simulink model "stepRecovery"  (Simulink 8.7)
settings: Solver=FixedStepDiscrete  StartTime=0.0  StopTime="CONFIG.SIMULATION_TIME "  FixedStep=CONFIG.Ts  RelTol=1e-3
InitFcn:
  | cd(fileparts(which(bdroot)));
  | initStepRecovery;
values from neighbouring files (symbols this model uses):
  baseToWorldRotationPort = '/matlabTorqueBalancing/floatingBaseRotationMatrix:i'    [esperimento_fake2.mat]    (also in initStepRecovery.m = ['/' WBT_modelName '/floatingBaseRotationMatrix:i']; initTorqueBalancing.m = ['/' WBT_modelName '/floatingBaseRotationMatrix:i']; secondo_risultato.mat)
  bVectorConstraints = [0 0 0 0 0 0 0 0 0 0 0 0 ... (19 elements, 19x1)]    [esperimento_fake2.mat]    (also in secondo_risultato.mat)
  CONFIG =     [esperimento_fake2.mat]    (also in secondo_risultato.mat)
  ConstraintsMatrix = [3.73205080757 1 0.267949192431 -0.267949192431 -1 -3.73205080757 -3.73205080757 -1 -0.267949192431 0.267949192431 1 3.73205080757 ... (114 elements, 19x6)]    [esperimento_fake2.mat]    (also in secondo_risultato.mat)
  gain =     [esperimento_fake2.mat]    (also in secondo_risultato.mat)
  references =     [esperimento_fake2.mat]    (also in secondo_risultato.mat)
  reg =     [esperimento_fake2.mat]    (also in secondo_risultato.mat)
  ROBOT_DOF = 23    [esperimento_fake2.mat]    (also in secondo_risultato.mat)
  ROBOT_DOF_FOR_SIMULINK = [1 0 0 0 0 0 0 0 0 0 0 0 ... (529 elements, 23x23)]    [esperimento_fake2.mat]    (also in secondo_risultato.mat)
  sat =     [esperimento_fake2.mat]    (also in secondo_risultato.mat)
  SM =     [esperimento_fake2.mat]    (also in secondo_risultato.mat)
  sm =     [esperimento_fake2.mat]    (also in secondo_risultato.mat)
  WBT_modelName = 'matlabTorqueBalancing'    [esperimento_fake2.mat]    (also in initStepRecovery.m; initTorqueBalancing.m; secondo_risultato.mat)
  WBT_robotName = ''    [esperimento_fake2.mat]    (also in secondo_risultato.mat)
undefined symbols (not defined in the file or in its folder): DiscIntNeverNeededParam
libraries: WBToolboxLibrary x171, simulink x16, simulink_extras x4
(part 4 of 5)

== system stepRecovery/DesValues/State Machine Step Recovery/visualise inertial/w_H_root_link4 ==
  qj : Inport
  inertial : Inport  Port=2
  "CoM6D ->  CoMXYZ1" : Selector  NumberOfDimensions=2  InputPortWidth=7  IndexOptions=Index vector (dialog),Index vector (dialog)  Indices=[1 2 3],[1 2 3]  OutputSizes=1,1
  Constant : Constant  Value=zeros(3,1)
  Constant2 : Constant  Value=eye(4)
  Constant5 : Constant  Value=eye(4)
  Constant6 : Constant  Value=eye(4)
  Gain : Gain  Gain=pi/180
  Head state : WBToolboxLibrary/Utilities/Yarp Read  portName=[WBT_robotName, '/head/state:o']  signalSize=6  blocking=off  timestamp=off  autoconnect=on  errorOnConnection=off
  Inv\* : Product  Inputs=/*  Multiplication=Matrix(*)
  Inv\*1 : Product  Inputs=/*  Multiplication=Matrix(*)
  Inv\*2 : Product  Inputs=/  Multiplication=Matrix(*)
  Product : Product  Multiplication=Matrix(*)
  Selector : Selector  InputPortWidth=12  IndexOptions=Index vector (dialog)  Indices=[4 5 6 ]  OutputSizes=1
  Selector1 : Selector  InputPortWidth=6  IndexOptions=Index vector (dialog)  Indices=[1:3]  OutputSizes=1
  Switch : Switch  Criteria=u2 > Threshold
  Switch6 : Switch  Criteria=u2 > Threshold
  USE_IMU4EST_BASE : Constant  Value=CONFIG.USE_IMU4EST_BASE
  USE_IMU4EST_BASE1 : Constant  Value=CONFIG.CORRECT_NECK_IMU
  fromImuToHomogeousTransformFCN : MATLAB Function  TreatAsAtomicUnit=on
  holder 1 : WBToolboxLibrary/Utilities/holder 
  holder 2 : WBToolboxLibrary/Utilities/holder 
  imu : WBToolboxLibrary/wholeBodyModel/Kinematics/Forward Kinematics  frameName='imu_frame'  robotName=WBT_robotName  localName=WBT_modelName  wbiFile=WBT_wbiFilename  wbiList=WBT_wbiList
  l_sole_acc : Scope
  link : WBToolboxLibrary/wholeBodyModel/Kinematics/Forward Kinematics  frameName=link_name  robotName=WBT_robotName  localName=WBT_modelName  wbiFile=WBT_wbiFilename  wbiList=WBT_wbiList
  root_link : WBToolboxLibrary/wholeBodyModel/Kinematics/Forward Kinematics  frameName='root_link'  robotName=WBT_robotName  localName=WBT_modelName  wbiFile=WBT_wbiFilename  wbiList=WBT_wbiList
  w_H_root : Outport
  wires:
  Constant/1 -> Switch/3
  Gain/1 -> Selector1/1
  Switch/1 -> fromImuToHomogeousTransformFCN/6(neck)
  USE_IMU4EST_BASE1/1 -> Switch/2
  Selector1/1 -> Switch/1  "neck"
  Head state/1 -> Gain/1
  Product/1 -> l_sole_acc/1
  Selector/1 -> Product/2  "imu_acce"
  "CoM6D ->  CoMXYZ1"/1 -> Product/1  "l_sole_R_imu"
  Inv\*2/1 -> "CoM6D ->  CoMXYZ1"/1
  holder 2/1 -> fromImuToHomogeousTransformFCN/4(inertial_0)
  holder 1/1 -> fromImuToHomogeousTransformFCN/2(imu_H_link_0)
  root_link/1 -> Inv\*1/2
  qj/1 -> imu/2, link/2, root_link/2
  Constant2/1 -> root_link/1
  fromImuToHomogeousTransformFCN/1(w_H_root) -> Switch6/1
  USE_IMU4EST_BASE/1 -> Switch6/2
  Switch6/1 -> w_H_root/1
  inertial/1 -> fromImuToHomogeousTransformFCN/5(inertial), holder 2/1, Selector/1
  link/1 -> Inv\*1/1, Inv\*/2
  Inv\*1/1 -> fromImuToHomogeousTransformFCN/3(link_H_root), Switch6/3  "link_H_root"
  Constant6/1 -> link/1
  imu/1 -> Inv\*/1
  Inv\*/1 -> fromImuToHomogeousTransformFCN/1(imu_H_link), holder 1/1, Inv\*2/1  "imu_H_link"
  Constant5/1 -> imu/1

== system stepRecovery/DesValues/State Machine/visualise inertial/l_sole_H_root_link2/Visualize hom transf4 ==
  H : Inport
  "CoM6D ->  CoMXYZ1" : Selector  NumberOfDimensions=2  InputPortWidth=7  IndexOptions=Index vector (dialog),Index vector (dialog)  Indices=[1 2 3],[1 2 3]  OutputSizes=1,1
  "CoM6D ->  CoMXYZ2" : Selector  NumberOfDimensions=2  InputPortWidth=7  IndexOptions=Index vector (dialog),Index vector (dialog)  Indices=[1 2 3],[4]  OutputSizes=1,1
  Hom : Scope
  R : Scope
  p : Scope
  wires:
  "CoM6D ->  CoMXYZ1"/1 -> R/1
  "CoM6D ->  CoMXYZ2"/1 -> p/1
  H/1 -> "CoM6D ->  CoMXYZ2"/1, Hom/1, "CoM6D ->  CoMXYZ1"/1

== system stepRecovery/DesValues/State Machine/visualise inertial/l_sole_H_root_link3/Visualize hom transf4 ==
  H : Inport
  "CoM6D ->  CoMXYZ1" : Selector  NumberOfDimensions=2  InputPortWidth=7  IndexOptions=Index vector (dialog),Index vector (dialog)  Indices=[1 2 3],[1 2 3]  OutputSizes=1,1
  "CoM6D ->  CoMXYZ2" : Selector  NumberOfDimensions=2  InputPortWidth=7  IndexOptions=Index vector (dialog),Index vector (dialog)  Indices=[1 2 3],[4]  OutputSizes=1,1
  Hom : Scope
  R : Scope
  p : Scope
  wires:
  "CoM6D ->  CoMXYZ1"/1 -> R/1
  "CoM6D ->  CoMXYZ2"/1 -> p/1
  H/1 -> "CoM6D ->  CoMXYZ2"/1, Hom/1, "CoM6D ->  CoMXYZ1"/1

== system stepRecovery/DesValues/State Machine Step Recovery/Step Recovery reference generator/Inverse Kinematics/Local inverse kin ==
  Desired Transformation : Inport
  w_H_b : Inport  Port=2
  qj : Inport  Port=3
  23-DoFs WBI to YARP : WBToolboxLibrary/Utilities/23-DoFs WBI to YARP
  Inverse Kinematics : WBToolboxLibrary/wholeBodyModel/Kinematics/Inverse Kinematics  baseFrame='l_sole'  endEffFrame='r_sole'  optOption=Full Constraint (Position and Orientation)  robotName=WBT_robotName  localName=WBT_modelName  wbiFile=WBT_wbiFilename  wbiList=WBT_wbiList
  Mux : Mux  Inputs=2
  Terminator{,1..3} (4 alike) : Terminator
  q_legs : Outport
  "q_total " : Outport  Port=2
  wires:
  Desired Transformation/1 -> Inverse Kinematics/1
  23-DoFs WBI to YARP/3 -> Terminator3/1
  Mux/1 -> q_legs/1
  w_H_b/1 -> Inverse Kinematics/2
  23-DoFs WBI to YARP/1 -> Terminator1/1
  23-DoFs WBI to YARP/2 -> Terminator2/1
  qj/1 -> Inverse Kinematics/3
  Inverse Kinematics/1 -> Terminator/1
  Inverse Kinematics/2 -> "q_total "/1, 23-DoFs WBI to YARP/1
  23-DoFs WBI to YARP/4 -> Mux/1
  23-DoFs WBI to YARP/5 -> Mux/2

== system stepRecovery/DesValues/State Machine Step Recovery/Step Recovery reference generator/Inverse Kinematics/Remote Inverse Kineamtics ==
  Desired Transformation : Inport
  q(0) : Inport  Port=2
  23-DoFs WBI to YARP1 : WBToolboxLibrary/Utilities/23-DoFs WBI to YARP
  Mux : Mux
  Mux2 : Mux  Inputs=2
  Remote Inverse Kinematics : WBToolboxLibrary/wholeBodyModel/Kinematics/Remote Inverse Kinematics  solverName='/cartesianSolver'  dofs=12  optOption=Full Constraint (Position and Orientation)
  Selector : Selector  InputPortWidth=6  IndexOptions=Index vector (dialog)  Indices=[6 5 4 3 2 1]  OutputSizes=1
  Selector1 : Selector  InputPortWidth=12  IndexOptions=Index vector (dialog)  Indices=[6, 5, 4, 3, 2, 1, 7:12]  OutputSizes=1
  q_legs : Outport
  q_total : Outport  Port=2
  wires:
  Desired Transformation/1 -> Remote Inverse Kinematics/1
  q(0)/1 -> 23-DoFs WBI to YARP1/1
  23-DoFs WBI to YARP1/5 -> Mux2/2
  Mux2/1 -> Remote Inverse Kinematics/2
  23-DoFs WBI to YARP1/4 -> Selector/1
  Selector/1 -> Mux2/1
  Selector1/1 -> Mux/4, q_legs/1
  Remote Inverse Kinematics/1 -> Selector1/1
  23-DoFs WBI to YARP1/1 -> Mux/1
  23-DoFs WBI to YARP1/2 -> Mux/2
  23-DoFs WBI to YARP1/3 -> Mux/3
  Mux/1 -> q_total/1

== system stepRecovery/DesValues/State Machine Step Recovery/Step Recovery reference generator/Step Recovery Techniques /Capture Point Computer ==
  r_Cxp : Inport
  COM velocity : Inport  Port=2
  COMx : Inport  Port=3
  w_H_lsole : Inport  Port=4
  w_H_rsole : Inport  Port=5
  "Constraints " : Inport  Port=6
  STATE : Inport  Port=7
  Capture Point : Subsystem
  Capture Point-alternative : Subsystem
  "ICP " : Subsystem
  Out of left foot_CH : Subsystem
  r_CP : Outport
  r_CP1 : Outport  Port=2
  OUT : Outport  Port=3
  Direction : Outport  Port=4
  OUT_REAL : Outport  Port=5
  OUT_CH : Outport  Port=6
  wires:
  r_Cxp/1 -> Capture Point-alternative/2(r_CxP), Capture Point/2(r_CxP)
  COMx/1 -> "ICP "/1(COM position), Capture Point-alternative/3(COMx), Capture Point/3(COMx)
  COM velocity/1 -> "ICP "/2(COM velocity)
  Capture Point/1("r_CP ") -> r_CP/1
  "ICP "/1(icp) -> Out of left foot_CH/1(X_global), Capture Point-alternative/4(r_icp), Capture Point/4(r_icp)
  Out of left foot_CH/1(OUT_L) -> Capture Point-alternative/5(OUT), Capture Point/5(OUT)
  Capture Point/2("STEP ") -> OUT/1
  Capture Point-alternative/1("r_CP ") -> r_CP1/1
  Capture Point/3(Direction) -> Direction/1
  Out of left foot_CH/2(OUT_CH) -> Capture Point-alternative/6(OUT_CH), Capture Point/6(OUT_CH), OUT_CH/1
  "Constraints "/1 -> Out of left foot_CH/2(Constraints)
  Out of left foot_CH/3(OUT_REAL) -> OUT_REAL/1
  w_H_lsole/1 -> Out of left foot_CH/3(w_H_lsole)
  w_H_rsole/1 -> Out of left foot_CH/4(w_H_rsole)
  STATE/1 -> Capture Point-alternative/1(STATE), Capture Point/1(STATE)

== system stepRecovery/DesValues/State Machine Step Recovery/Step Recovery reference generator/Step Recovery Techniques /Dump and Visualize SRT  ==
  w_H_b : Inport
  COP : Inport  Port=2
  CMP : Inport  Port=3
  com_lin_vel : Inport  Port=4
  nu : Inport  Port=5
  CP : Inport  Port=6
  CP1 : Inport  Port=7
  TRIGGER CP : Inport  Port=8
  OUT_REAL_CP : Inport  Port=9
  CH_CP : Inport  Port=10
  FPE : Inport  Port=11
  TRIGGER FPE : Inport  Port=12
  FPE ORIGINAL : Inport  Port=13
  theta_bar : Inport  Port=14
  OUT_REAL_FPE : Inport  Port=15
  CH_FPE : Inport  Port=16
  CH_CP_dup : InportShadow  Port=10
  CH_FPE_dup : InportShadow  Port=16
  CP1_dup : InportShadow  Port=7
  CP_dup : InportShadow  Port=6
  FPE_dup : InportShadow  Port=11
  Subsystem : Subsystem
  TRIGGER CP_dup : InportShadow  Port=8
  TRIGGER FPE_dup : InportShadow  Port=12
  "Visualize " : Subsystem
  wires:
  w_H_b/1 -> Subsystem/1(w_H_b)
  COP/1 -> Subsystem/2(COP)
  CMP/1 -> Subsystem/3(CMP)
  com_lin_vel/1 -> Subsystem/4(com_lin_vel)
  nu/1 -> Subsystem/5(nu)
  CP_dup/1 -> Subsystem/6(CP)
  CP1_dup/1 -> Subsystem/7(CP1)
  TRIGGER CP_dup/1 -> Subsystem/8(TRIGGER CP)
  CH_CP_dup/1 -> Subsystem/9(CH_CP)
  FPE_dup/1 -> Subsystem/10(FPE)
  TRIGGER FPE_dup/1 -> Subsystem/11(TRIGGER FPE)
  CH_FPE_dup/1 -> Subsystem/12(CH_FPE)
  CP/1 -> "Visualize "/1(CP)
  CP1/1 -> "Visualize "/2(CP1)
  TRIGGER CP/1 -> "Visualize "/3(TRIGGER CP)
  OUT_REAL_CP/1 -> "Visualize "/4(OUT_REAL_CP)
  CH_CP/1 -> "Visualize "/5(CH_CP)
  FPE/1 -> "Visualize "/6(FPE)
  TRIGGER FPE/1 -> "Visualize "/7(TRIGGER FPE)
  FPE ORIGINAL/1 -> "Visualize "/8(FPE ORIGINAL)
  theta_bar/1 -> "Visualize "/9(theta_bar)
  OUT_REAL_FPE/1 -> "Visualize "/10(OUT_REAL_FPE)
  CH_FPE/1 -> "Visualize "/11(CH_FPE)

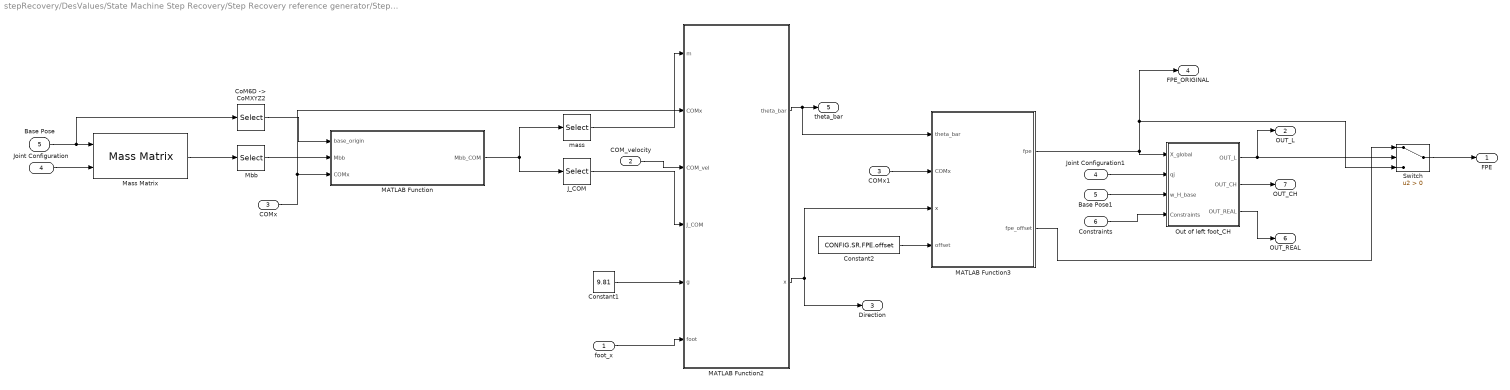
== system stepRecovery/DesValues/State Machine Step Recovery/Step Recovery reference generator/Step Recovery Techniques /FPE module ==
  foot_x : Inport
  COM_velocity : Inport  Port=2
  COMx : Inport  Port=3
  Joint Configuration : Inport  Port=4
  Base Pose : Inport  Port=5
  Constraints : Inport  Port=6
  Base Pose1 : InportShadow  Port=5
  COMx1 : InportShadow  Port=3
  "CoM6D ->  CoMXYZ2" : Selector  NumberOfDimensions=2  InputPortWidth=7  IndexOptions=Index vector (dialog),Index vector (dialog)  Indices=[1 2 3],[4]  OutputSizes=1,1
  Constant1 : Constant  Value=9.81
  Constant2 : Constant  Value=CONFIG.SR.FPE.offset
  J_COM : Selector  NumberOfDimensions=2  InputPortWidth=3  IndexOptions=Index vector (dialog),Index vector (dialog)  Indices=[4:6],[4:6]  OutputSizes=1,1
  Joint Configuration1 : InportShadow  Port=4
  MATLAB Function : MATLAB Function  TreatAsAtomicUnit=on
  MATLAB Function2 : MATLAB Function  TreatAsAtomicUnit=on
  MATLAB Function3 : MATLAB Function  TreatAsAtomicUnit=on
  Mass Matrix : WBToolboxLibrary/wholeBodyModel/Dynamics/Mass Matrix  robotName=WBT_robotName  localName=WBT_modelName  wbiFile=WBT_wbiFilename  wbiList=WBT_wbiList
  Mbb : Selector  NumberOfDimensions=2  InputPortWidth=3  IndexOptions=Index vector (dialog),Index vector (dialog)  Indices=[1:6],[1:6]  OutputSizes=1,1
  Out of left foot_CH : Subsystem
  Switch : Switch  Criteria=u2 > Threshold
  mass : Selector  NumberOfDimensions=2  InputPortWidth=3  IndexOptions=Index vector (dialog),Index vector (dialog)  Indices=[1],[1]  OutputSizes=1,1
  FPE : Outport
  OUT_L : Outport  Port=2
  Direction : Outport  Port=3
  FPE_ORIGINAL : Outport  Port=4
  theta_bar : Outport  Port=5
  OUT_REAL : Outport  Port=6
  OUT_CH : Outport  Port=7
  wires:
  Mass Matrix/1 -> Mbb/1
  Base Pose/1 -> "CoM6D ->  CoMXYZ2"/1, Mass Matrix/1
  Joint Configuration/1 -> Mass Matrix/2
  Mbb/1 -> MATLAB Function/2(Mbb)
  MATLAB Function/1(Mbb_COM) -> J_COM/1, mass/1
  "CoM6D ->  CoMXYZ2"/1 -> MATLAB Function/1(base_origin)
  COM_velocity/1 -> MATLAB Function2/3(COM_vel)
  mass/1 -> MATLAB Function2/1(m)
  J_COM/1 -> MATLAB Function2/4(J_COM)
  COMx/1 -> MATLAB Function2/2(COMx), MATLAB Function/3(COMx)
  Constant1/1 -> MATLAB Function2/5(g)
  MATLAB Function2/1(theta_bar) -> MATLAB Function3/1(theta_bar), theta_bar/1
  foot_x/1 -> MATLAB Function2/6(foot)
  MATLAB Function2/2(x) -> MATLAB Function3/3(x), Direction/1
  Constant2/1 -> MATLAB Function3/4(offset)
  COMx1/1 -> MATLAB Function3/2(COMx)
  MATLAB Function3/1(fpe) -> Out of left foot_CH/1(X_global), Switch/3, FPE_ORIGINAL/1
  Base Pose1/1 -> Out of left foot_CH/3(w_H_base)
  Joint Configuration1/1 -> Out of left foot_CH/2(qj)
  Constraints/1 -> Out of left foot_CH/4(Constraints)
  Out of left foot_CH/1(OUT_L) -> Switch/2, OUT_L/1
  Out of left foot_CH/2(OUT_CH) -> OUT_CH/1
  Out of left foot_CH/3(OUT_REAL) -> OUT_REAL/1
  MATLAB Function3/2(fpe_offset) -> Switch/1
  Switch/1 -> FPE/1

== system stepRecovery/DesValues/State Machine Step Recovery/Step Recovery reference generator/Step Recovery Techniques /ankle, CoP, Cmp (LEFT FOOT) ==
  Contact_Wrench : Inport
  CoMx : Inport  Port=2
  w_H_lsole : Inport  Port=3
  CMP computer : Subsystem
  COP computer : Subsystem
  Constant : Constant
  Matrix Multiply : Product  Multiplication=Matrix(*)
  Mux1 : Mux  Inputs=2
  Selector : Selector  NumberOfDimensions=2  InputPortWidth=3  IndexOptions=Index vector (dialog),Index vector (dialog)  Indices=[1: 3],4  OutputSizes=1,1
  Selector1 : Selector  InputPortWidth=4  IndexOptions=Index vector (dialog)  Indices=[1:3]  OutputSizes=1
  Sum1 : Sum  Inputs=-+|
  xAnkle : Outport
  CoP : Outport  Port=2
  deltaCoP : Outport  Port=3
  r_CMP : Outport  Port=4
  deltaCMP : Outport  Port=5
  wires:
  Constant/1 -> Mux1/2
  w_H_lsole/1 -> CMP computer/1(w_H_l), Matrix Multiply/1, Selector/1
  Mux1/1 -> Matrix Multiply/2
  Matrix Multiply/1 -> Selector1/1
  COP computer/1(DeltaR_Cop) -> deltaCoP/1, Mux1/1
  Selector/1 -> Sum1/1, xAnkle/1
  Selector1/1 -> CoP/1
  Contact_Wrench/1 -> CMP computer/2(Contact Wrench), COP computer/1(Contact Wrench)
  CMP computer/1(R_CMP) -> r_CMP/1, Sum1/2
  Sum1/1 -> deltaCMP/1
  CoMx/1 -> CMP computer/3(COM position)

== system stepRecovery/DesValues/State Machine Step Recovery/visualise inertial/l_sole_H_root_link2/Visualize hom transf4 ==
  H : Inport
  "CoM6D ->  CoMXYZ1" : Selector  NumberOfDimensions=2  InputPortWidth=7  IndexOptions=Index vector (dialog),Index vector (dialog)  Indices=[1 2 3],[1 2 3]  OutputSizes=1,1
  "CoM6D ->  CoMXYZ2" : Selector  NumberOfDimensions=2  InputPortWidth=7  IndexOptions=Index vector (dialog),Index vector (dialog)  Indices=[1 2 3],[4]  OutputSizes=1,1
  Hom : Scope
  R : Scope
  p : Scope
  wires:
  H/1 -> "CoM6D ->  CoMXYZ1"/1, Hom/1, "CoM6D ->  CoMXYZ2"/1
  "CoM6D ->  CoMXYZ2"/1 -> p/1
  "CoM6D ->  CoMXYZ1"/1 -> R/1

== system stepRecovery/DesValues/State Machine Step Recovery/visualise inertial/l_sole_H_root_link3/Visualize hom transf4 ==
  H : Inport
  "CoM6D ->  CoMXYZ1" : Selector  NumberOfDimensions=2  InputPortWidth=7  IndexOptions=Index vector (dialog),Index vector (dialog)  Indices=[1 2 3],[1 2 3]  OutputSizes=1,1
  "CoM6D ->  CoMXYZ2" : Selector  NumberOfDimensions=2  InputPortWidth=7  IndexOptions=Index vector (dialog),Index vector (dialog)  Indices=[1 2 3],[4]  OutputSizes=1,1
  Hom : Scope
  R : Scope
  p : Scope
  wires:
  H/1 -> "CoM6D ->  CoMXYZ1"/1, Hom/1, "CoM6D ->  CoMXYZ2"/1
  "CoM6D ->  CoMXYZ2"/1 -> p/1
  "CoM6D ->  CoMXYZ1"/1 -> R/1

== system stepRecovery/DesValues/State Machine Step Recovery/Step Recovery reference generator/Step Recovery Techniques /Capture Point Computer/Capture Point ==
  STATE : Inport
  r_CxP : Inport  Port=2
  COMx : Inport  Port=3
  r_icp : Inport  Port=4
  OUT : Inport  Port=5
  OUT_CH : Inport  Port=6
  Compare To Constant : simulink/Logic and Bit Operations/Compare To Constant  relop===  const=14  OutDataTypeStr=boolean
  Constant : Constant  Value=CONFIG.Ts
  Constant1 : Constant  Value=CONFIG.SR.CP.robotStepTime
  Data Type Conversion : DataTypeConversion  OutDataTypeStr=boolean
  Data Type Conversion2 : DataTypeConversion  OutDataTypeStr=double
  Logical Operator : Logic  Operator=NOR  AllPortsSameDT=off  OutDataTypeStr=boolean
  MATLAB Function : MATLAB Function  TreatAsAtomicUnit=on
  MATLAB Function1 : MATLAB Function  TreatAsAtomicUnit=on
  S-R Flip-Flop : simulink_extras/Flip Flops/S-R Flip-Flop  initial_condition=0
  Versor : MATLAB Function  TreatAsAtomicUnit=on
  omega : Subsystem
  "r_CP " : Outport
  "STEP " : Outport  Port=2
  Direction : Outport  Port=3
  wires:
  Data Type Conversion/1 -> S-R Flip-Flop/1
  r_CxP/1 -> Versor/1(r_CxP), MATLAB Function1/2(r)
  S-R Flip-Flop/1 -> Data Type Conversion2/1
  omega/1(omega) -> Versor/2(omega), MATLAB Function/1(omega), MATLAB Function1/1(omega)
  Constant/1 -> MATLAB Function1/3(delta_t)
  COMx/1 -> omega/1(COMx)
  MATLAB Function1/1(r_eq) -> MATLAB Function/3(r_CxP)
  Constant1/1 -> MATLAB Function/4(robot_step_time)
  MATLAB Function/1(r_CP) -> "r_CP "/1
  Data Type Conversion2/1 -> "STEP "/1, MATLAB Function/5(STEP), MATLAB Function1/4(OUT)
  r_icp/1 -> Versor/3(r_ic), MATLAB Function/2(r_ic)
  Versor/1(direction) -> Direction/1
  Logical Operator/1 -> S-R Flip-Flop/2
  OUT/1 -> Data Type Conversion/1
  STATE/1 -> Compare To Constant/1
  Compare To Constant/1 -> Logical Operator/2
  OUT_CH/1 -> Logical Operator/1

== system stepRecovery/DesValues/State Machine Step Recovery/Step Recovery reference generator/Step Recovery Techniques /Capture Point Computer/Capture Point-alternative ==
  STATE : Inport
  r_CxP : Inport  Port=2
  COMx : Inport  Port=3
  r_icp : Inport  Port=4
  OUT : Inport  Port=5
  OUT_CH : Inport  Port=6
  Compare To Constant : simulink/Logic and Bit Operations/Compare To Constant  relop===  const=14  OutDataTypeStr=boolean
  Constant1 : Constant  Value=CONFIG.SR.CP.robotStepTime
  Constant2 : Constant  Value=CONFIG.Ts
  Data Type Conversion : DataTypeConversion  OutDataTypeStr=boolean
  Data Type Conversion2 : DataTypeConversion  OutDataTypeStr=double
  Logical Operator : Logic  Operator=NOR  AllPortsSameDT=off  OutDataTypeStr=boolean
  MATLAB Function : MATLAB Function  TreatAsAtomicUnit=on
  S-R Flip-Flop : simulink_extras/Flip Flops/S-R Flip-Flop  initial_condition=0
  omega : Subsystem
  "r_CP " : Outport
  "STEP " : Outport  Port=2
  wires:
  Constant2/1 -> MATLAB Function/6(delta_t)
  Data Type Conversion2/1 -> MATLAB Function/5(STEP), "STEP "/1
  MATLAB Function/1(r_CP) -> "r_CP "/1
  Constant1/1 -> MATLAB Function/4(robot_step_time)
  r_icp/1 -> MATLAB Function/2(r_ic)
  r_CxP/1 -> MATLAB Function/3(r_CxP)
  COMx/1 -> omega/1(COMx)
  omega/1(omega) -> MATLAB Function/1(omega)
  S-R Flip-Flop/1 -> Data Type Conversion2/1
  Data Type Conversion/1 -> S-R Flip-Flop/1
  OUT/1 -> Data Type Conversion/1
  Logical Operator/1 -> S-R Flip-Flop/2
  OUT_CH/1 -> Logical Operator/1
  STATE/1 -> Compare To Constant/1
  Compare To Constant/1 -> Logical Operator/2

== system stepRecovery/DesValues/State Machine Step Recovery/Step Recovery reference generator/Step Recovery Techniques /Capture Point Computer/ICP  ==
  note: Instantaneous capture point
  COM position : Inport
  COM velocity : Inport  Port=2
  Divide1 : Product  Inputs=/*
  Sum : Sum  Inputs=|++
  omega : Subsystem
  zero height : Gain  Gain=[1,0,0;0,1,0;0,0,0]  Multiplication=Matrix(K*u)
  icp : Outport
  wires:
  COM position/1 -> omega/1(COMx), Sum/1
  Divide1/1 -> Sum/2
  COM velocity/1 -> Divide1/2
  Sum/1 -> zero height/1
  zero height/1 -> icp/1
  omega/1(omega) -> Divide1/1

== system stepRecovery/DesValues/State Machine Step Recovery/Step Recovery reference generator/Step Recovery Techniques /Capture Point Computer/Out of left foot_CH ==
  X_global : Inport
  Constraints : Inport  Port=2
  w_H_lsole : Inport  Port=3
  w_H_rsole : Inport  Port=4
  Constant : Constant
  Constant1 : Constant  Value=gain.l_foot_shadowed
  Constant2 : Constant  Value=gain.footSize_step
  Constant3 : Constant  Value=gain.footSize
  Inverse : MATLAB Function  TreatAsAtomicUnit=on
  MATLAB Function : MATLAB Function  TreatAsAtomicUnit=on
  Matrix Multiply : Product  Multiplication=Matrix(*)
  Mux : Mux  Inputs=2
  "Out of left foot " : MATLAB Function  TreatAsAtomicUnit=on
  Selector : Selector  InputPortWidth=2  IndexOptions=Index vector (dialog)  Indices=[2]  OutputSizes=1
  Selector2 : Selector  InputPortWidth=4  IndexOptions=Index vector (dialog)  Indices=[1 2]  OutputSizes=1
  Switch : Switch  Criteria=u2 > Threshold
  OUT_L : Outport
  OUT_CH : Outport  Port=2
  OUT_REAL : Outport  Port=3
  wires:
  Mux/1 -> Matrix Multiply/2
  Selector2/1 -> "Out of left foot "/1(x)
  Matrix Multiply/1 -> Selector2/1
  Constant/1 -> Mux/2
  w_H_lsole/1 -> MATLAB Function/2(w_H_lsole), Inverse/1(w_H_a)
  "Out of left foot "/1(OUT) -> Switch/3, OUT_L/1
  X_global/1 -> MATLAB Function/1(x), Mux/1
  Inverse/1(a_H_w) -> Matrix Multiply/1
  Constant2/1 -> "Out of left foot "/2(support)
  Constant1/1 -> "Out of left foot "/3(shadow)
  Constant3/1 -> MATLAB Function/4(foot_size)
  w_H_rsole/1 -> MATLAB Function/3(w_H_rsole)
  MATLAB Function/1(OUT) -> Switch/1
  Constraints/1 -> Selector/1
  Selector/1 -> Switch/2
  Switch/1 -> OUT_CH/1
  "Out of left foot "/2(OUT_real) -> OUT_REAL/1

== system stepRecovery/DesValues/State Machine Step Recovery/Step Recovery reference generator/Step Recovery Techniques /Dump and Visualize SRT /Subsystem ==
  w_H_b : Inport
  COP : Inport  Port=2
  CMP : Inport  Port=3
  com_lin_vel : Inport  Port=4
  nu : Inport  Port=5
  CP : Inport  Port=6
  CP1 : Inport  Port=7
  TRIGGER CP : Inport  Port=8
  CH_CP : Inport  Port=9
  FPE : Inport  Port=10
  TRIGGER FPE : Inport  Port=11
  CH_FPE : Inport  Port=12
  To Workspace : ToWorkspace  VariableName=nu  SampleTime=-1
  To Workspace1 : ToWorkspace  VariableName=COM_lin_vel  SampleTime=-1
  To Workspace10 : ToWorkspace  VariableName=OUT_CONVEXHULL_CP  SampleTime=-1
  To Workspace11 : ToWorkspace  VariableName=OUT_CONVEXHULL_FPE  SampleTime=-1
  To Workspace2 : ToWorkspace  VariableName=w_H_b  SampleTime=-1
  To Workspace3 : ToWorkspace  VariableName=CMP  SampleTime=-1
  To Workspace4 : ToWorkspace  VariableName=COP  SampleTime=-1
  To Workspace5 : ToWorkspace  VariableName=FPE  SampleTime=-1
  To Workspace6 : ToWorkspace  VariableName=TRIGGER_FPE  SampleTime=-1
  To Workspace7 : ToWorkspace  VariableName=TRIGGER_CP  SampleTime=-1
  To Workspace8 : ToWorkspace  VariableName=CP  SampleTime=-1
  To Workspace9 : ToWorkspace  VariableName=CP1  SampleTime=-1
  wires:
  COP/1 -> To Workspace4/1
  com_lin_vel/1 -> To Workspace1/1
  CMP/1 -> To Workspace3/1
  w_H_b/1 -> To Workspace2/1
  nu/1 -> To Workspace/1
  FPE/1 -> To Workspace5/1
  CP/1 -> To Workspace8/1
  CH_CP/1 -> To Workspace10/1
  CH_FPE/1 -> To Workspace11/1
  CP1/1 -> To Workspace9/1
  TRIGGER CP/1 -> To Workspace7/1
  TRIGGER FPE/1 -> To Workspace6/1

== system stepRecovery/DesValues/State Machine Step Recovery/Step Recovery reference generator/Step Recovery Techniques /Dump and Visualize SRT /Visualize  ==
  CP : Inport
  CP1 : Inport  Port=2
  TRIGGER CP : Inport  Port=3
  OUT_REAL_CP : Inport  Port=4
  CH_CP : Inport  Port=5
  FPE : Inport  Port=6
  TRIGGER FPE : Inport  Port=7
  FPE ORIGINAL : Inport  Port=8
  theta_bar : Inport  Port=9
  OUT_REAL_FPE : Inport  Port=10
  CH_FPE : Inport  Port=11
  FPE_1 : InportShadow  Port=6
  Mux : Mux  Inputs=3
  Mux2 : Mux  Inputs=3
  Scope1 : Scope  Commented=on  NumInputPorts=4
  Scope2 : Scope  NumInputPorts=4
  Scope3 : Scope  Commented=on  NumInputPorts=2
  TRIGGER FPE_1 : InportShadow  Port=7
  wires:
  TRIGGER CP/1 -> Scope3/1, Mux/1
  CP/1 -> Scope2/1
  FPE/1 -> Scope2/3
  CP1/1 -> Scope2/2
  TRIGGER FPE/1 -> Mux/3
  CH_CP/1 -> Mux/2
  CH_FPE/1 -> Mux2/3
  OUT_REAL_CP/1 -> Scope3/2
  FPE ORIGINAL/1 -> Scope1/2
  theta_bar/1 -> Scope1/3
  Mux2/1 -> Scope1/4  "Triggers"
  OUT_REAL_FPE/1 -> Mux2/2
  Mux/1 -> Scope2/4  "Triggers"
  FPE_1/1 -> Scope1/1
  TRIGGER FPE_1/1 -> Mux2/1

== system stepRecovery/DesValues/State Machine Step Recovery/Step Recovery reference generator/Step Recovery Techniques /FPE module/Out of left foot_CH ==
  X_global : Inport
  qj : Inport  Port=2
  w_H_base : Inport  Port=3
  Constraints : Inport  Port=4
  Constant : Constant
  Constant1 : Constant  Value=gain.l_foot_shadowed
  Constant2 : Constant  Value=gain.footSize_step
  Constant3 : Constant  Value=gain.footSize
  Forward Kinematics1 : WBToolboxLibrary/wholeBodyModel/Kinematics/Forward Kinematics  frameName='l_sole'  robotName=WBT_robotName  localName=WBT_modelName  wbiFile=WBT_wbiFilename  wbiList=WBT_wbiList
  Forward Kinematics2 : WBToolboxLibrary/wholeBodyModel/Kinematics/Forward Kinematics  frameName='l_sole'  robotName=WBT_robotName  localName=WBT_modelName  wbiFile=WBT_wbiFilename  wbiList=WBT_wbiList
  Inverse : MATLAB Function  TreatAsAtomicUnit=on
  MATLAB Function : MATLAB Function  TreatAsAtomicUnit=on
  Matrix Multiply : Product  Multiplication=Matrix(*)
  Mux : Mux  Inputs=2
  "Out of left foot " : MATLAB Function  TreatAsAtomicUnit=on
  Selector : Selector  InputPortWidth=2  IndexOptions=Index vector (dialog)  Indices=[2]  OutputSizes=1
  Selector2 : Selector  InputPortWidth=4  IndexOptions=Index vector (dialog)  Indices=[1 2]  OutputSizes=1
  Switch : Switch  Criteria=u2 > Threshold
  OUT_L : Outport
  OUT_CH : Outport  Port=2
  OUT_REAL : Outport  Port=3
  wires:
  Mux/1 -> Matrix Multiply/2
  w_H_base/1 -> Forward Kinematics2/1, Forward Kinematics1/1
  Selector2/1 -> "Out of left foot "/1(x)
  Matrix Multiply/1 -> Selector2/1
  Constant/1 -> Mux/2
  Forward Kinematics1/1 -> MATLAB Function/2(w_H_lsole), Inverse/1(w_H_a)
  qj/1 -> Forward Kinematics2/2, Forward Kinematics1/2
  "Out of left foot "/1(OUT) -> Switch/3, OUT_L/1
  X_global/1 -> MATLAB Function/1(x), Mux/1
  Inverse/1(a_H_w) -> Matrix Multiply/1
  Constant2/1 -> "Out of left foot "/2(support)
  Constant1/1 -> "Out of left foot "/3(shadow)
  Constant3/1 -> MATLAB Function/4(foot_size)
  Forward Kinematics2/1 -> MATLAB Function/3(w_H_rsole)
  MATLAB Function/1(OUT) -> Switch/1
  Constraints/1 -> Selector/1
  Selector/1 -> Switch/2
  Switch/1 -> OUT_CH/1
  "Out of left foot "/2(OUT_real) -> OUT_REAL/1

== system stepRecovery/DesValues/State Machine Step Recovery/Step Recovery reference generator/Step Recovery Techniques /ankle, CoP, Cmp (LEFT FOOT)/CMP computer ==
  note: expressed in global coordinates
  w_H_l : Inport
  Contact Wrench : Inport  Port=2
  COM position : Inport  Port=3
  Demux : Demux  Outputs=3
  Divide : Product  Inputs=*/
  Divide1 : Product  Inputs=*/
  MATLAB Function : MATLAB Function  TreatAsAtomicUnit=on
  Matrix Multiply : Product  Multiplication=Matrix(*)
  Mux : Mux  Inputs=3
  Product : Product
  Product1 : Product
  Selector : Selector  InputPortWidth=6  IndexOptions=Index vector (dialog)  Indices=[1:3]  OutputSizes=1
  Selector1 : Selector  InputPortWidth=3  IndexOptions=Index vector (dialog)  Indices=[3]  OutputSizes=1
  Selector2 : Selector  NumberOfDimensions=2  InputPortWidth=3  IndexOptions=Index vector (dialog),Index vector (dialog)  Indices=[1:3],1:3  OutputSizes=1,1
  Selector3 : Selector  NumberOfDimensions=2  InputPortWidth=3  IndexOptions=Index vector (dialog),Index vector (dialog)  Indices=[1:3],4  OutputSizes=1,1
  Sum : Sum  Inputs=+-|
  Transpose : PermuteDimensions
  R_CMP : Outport
  wires:
  Divide/1 -> Product/2
  Product/1 -> Mux/1
  Divide1/1 -> Product1/2
  Sum/1 -> R_CMP/1
  Selector/1 -> Demux/1
  Demux/1 -> Divide/1
  Demux/3 -> Divide/2, Divide1/2
  Demux/2 -> Divide1/1
  COM position/1 -> Sum/1, Selector1/1
  Product1/1 -> Mux/2
  Mux/1 -> Sum/2
  Selector1/1 -> Mux/3, Product1/1, Product/1
  w_H_l/1 -> Selector2/1, Selector3/1
  MATLAB Function/1(s_A_b) -> Transpose/1
  Selector2/1 -> MATLAB Function/1(R)
  Selector3/1 -> MATLAB Function/2(p)
  Matrix Multiply/1 -> Selector/1
  Transpose/1 -> Matrix Multiply/1
  Contact Wrench/1 -> Matrix Multiply/2

== system stepRecovery/DesValues/State Machine Step Recovery/Step Recovery reference generator/Step Recovery Techniques /ankle, CoP, Cmp (LEFT FOOT)/COP computer ==
  Contact Wrench : Inport
  Constant : Constant  Value=0
  Demux : Demux  Outputs=3
  Divide : Product  Inputs=*/
  Divide1 : Product  Inputs=*/
  Gain : Gain  Gain=-1
  Mux : Mux  Inputs=3
  Selector : Selector  InputPortWidth=6  IndexOptions=Index vector (dialog)  Indices=[3:5]  OutputSizes=1
  DeltaR_Cop : Outport
  wires:
  Demux/3 -> Divide/1
  Demux/1 -> Divide1/2, Divide/2
  Demux/2 -> Divide1/1
  Divide/1 -> Gain/1
  Gain/1 -> Mux/1
  Divide1/1 -> Mux/2
  Constant/1 -> Mux/3
  Mux/1 -> DeltaR_Cop/1
  Selector/1 -> Demux/1
  Contact Wrench/1 -> Selector/1

== system stepRecovery/DesValues/State Machine Step Recovery/Step Recovery reference generator/Step Recovery Techniques /Capture Point Computer/Capture Point/omega ==
  COMx : Inport
  Constant : Constant  Value=9.81
  Divide : Product  Inputs=*/
  Selector : Selector  InputPortWidth=3  IndexOptions=Index vector (dialog)  Indices=[3]  OutputSizes=1
  Sqrt : Sqrt  SaturateOnIntegerOverflow=on
  holder 1 : WBToolboxLibrary/Utilities/holder 
  omega : Outport
  wires:
  COMx/1 -> Selector/1
  Selector/1 -> holder 1/1
  holder 1/1 -> Divide/2
  Constant/1 -> Divide/1
  Divide/1 -> Sqrt/1
  Sqrt/1 -> omega/1

== system stepRecovery/DesValues/State Machine Step Recovery/Step Recovery reference generator/Step Recovery Techniques /Capture Point Computer/Capture Point-alternative/omega ==
  COMx : Inport
  Constant : Constant  Value=9.81
  Divide : Product  Inputs=*/
  Selector : Selector  InputPortWidth=3  IndexOptions=Index vector (dialog)  Indices=[3]  OutputSizes=1
  Sqrt : Sqrt  SaturateOnIntegerOverflow=on
  holder 1 : WBToolboxLibrary/Utilities/holder 
  omega : Outport
  wires:
  Sqrt/1 -> omega/1
  Divide/1 -> Sqrt/1
  Constant/1 -> Divide/1
  holder 1/1 -> Divide/2
  Selector/1 -> holder 1/1
  COMx/1 -> Selector/1

== system stepRecovery/DesValues/State Machine Step Recovery/Step Recovery reference generator/Step Recovery Techniques /Capture Point Computer/ICP /omega ==
  COMx : Inport
  Constant : Constant  Value=9.81
  Divide : Product  Inputs=*/
  Selector : Selector  InputPortWidth=3  IndexOptions=Index vector (dialog)  Indices=[3]  OutputSizes=1
  Sqrt : Sqrt  SaturateOnIntegerOverflow=on
  holder 1 : WBToolboxLibrary/Utilities/holder 
  omega : Outport
  wires:
  COMx/1 -> Selector/1
  Selector/1 -> holder 1/1
  holder 1/1 -> Divide/2
  Constant/1 -> Divide/1
  Divide/1 -> Sqrt/1
  Sqrt/1 -> omega/1

== matlab function DesValues/State Machine/visualise inertial/w_H_root_link1/fromImuToHomogeousTransformFCN ==
  data: imu_H_link input double; imu_H_link_0 input double; link_H_root input double; inertial_0 input double; inertial input double; neck input double; w_H_root output double; CONFIG parameter double
function w_H_root = fromBaseToWorldWithImuFCN(imu_H_link,imu_H_link_0,link_H_root,inertial_0,inertial,neck,CONFIG)
%#codegen
w_H_root = fromBaseToWorldWithImu(imu_H_link,imu_H_link_0,link_H_root,inertial_0,inertial,neck,CONFIG);

== matlab function DesValues/Internal coordinator/w_H_root_link4/fromImuToHomogeousTransformFCN ==
  data: imu_H_link input double; imu_H_link_0 input double; link_H_root input double; inertial_0 input double; inertial input double; neck input double; w_H_root output double; CONFIG parameter double
function w_H_root = fromBaseToWorldWithImuFCN(imu_H_link,imu_H_link_0,link_H_root,inertial_0,inertial,neck,CONFIG)
%#codegen
w_H_root = fromBaseToWorldWithImu(imu_H_link,imu_H_link_0,link_H_root,inertial_0,inertial,neck,CONFIG);

== matlab function DesValues/MATLAB Function ==
  data: w_H_b_vectorised input double; w_H_b output double; foot_p_b input double; rollPitchYaw output double
function [w_H_b,rollPitchYaw] = buildHomogenousTranformation(w_H_b_vectorised,foot_p_b)
%#codegen

w_H_b = [w_H_b_vectorised(1:4),w_H_b_vectorised(5:8),w_H_b_vectorised(9:12),...
         w_H_b_vectorised(13:16)];

w_H_b(1:3,4) = foot_p_b;
rollPitchYaw = rollPitchYawFromRotation(w_H_b(1:3,1:3));
rollPitchYaw(3) = 0;

== matlab function controller_QP/integralOf Hw/MATLAB Function ==
  data: qjErr input double; dqjEquivalent output double; Jc input double; vbEquivalent output double
function [dqjEquivalent, vbEquivalent] = generateReferencesForH(qjErr,Jc)
%#codegen

dqjEquivalent = qjErr;
vbEquivalent  = -eye(6)/Jc(1:6,1:6)*Jc(1:6,7:end)*qjErr;

end

== matlab function DesValues/State Machine Walking/nu/MATLAB Function ==
  data: JcLeftFoot input double; JcRightFoot input double; activeFeetConstraints input double; y output double; qD input double; reg parameter double
function y = fcn(JcLeftFoot,JcRightFoot,activeFeetConstraints,qD,reg)
%#codegen

Jc = [activeFeetConstraints(1)*JcLeftFoot;
      activeFeetConstraints(2)*JcRightFoot];

pinvJb = (Jc(:,1:6)'*Jc(:,1:6) + reg.pinvDampVb*eye(6))\Jc(:,1:6)';  
  
% pinvJb = pinv(Jc(:,1:6));

y = -pinvJb*Jc(:,7:end)*qD;

== matlab function DesValues/State Machine Walking/stateMachineFCN ==
  data: connection input double; wrench_rightFoot input double; wrench_leftFoot input double; CoM_0 input double; q0 input double; w_CoM input double; CoMIn input double; qIn input double; constraintsIn input double; w_H_b output double; CoMDes output double; qDes output double; constraints output double; l_sole_H_b input double; r_sole_H_b input double; sm parameter double; impedances output double; gain parameter double; currentState output double
function [w_H_b, CoMDes,qDes,constraints,impedances,currentState] = ...
    stateMachineFCN(connection,wrench_rightFoot,wrench_leftFoot,CoM_0, q0, w_CoM , CoMIn, qIn, constraintsIn, l_sole_H_b, r_sole_H_b, sm,gain)
%#codegen
 
[CoMDes,qDes,constraints, currentState,impedances,w_H_b] = ...
    stateMachineWalking(connection,CoM_0, q0, w_CoM, CoMIn, qIn, constraintsIn, wrench_rightFoot,wrench_leftFoot,l_sole_H_b, r_sole_H_b, sm,gain);

== matlab function DesValues/Internal coordinator/nu/MATLAB Function ==
  data: JcLeftFoot input double; JcRightFoot input double; activeFeetConstraints input double; y output double; qD input double; reg parameter double
function y = fcn(JcLeftFoot,JcRightFoot,activeFeetConstraints,qD,reg)
%#codegen

Jc = [activeFeetConstraints(1)*JcLeftFoot;
      activeFeetConstraints(2)*JcRightFoot];

pinvJb = (Jc(:,1:6)'*Jc(:,1:6) + reg.pinvDampVb*eye(6))\Jc(:,1:6)';  
  
% pinvJb = pinv(Jc(:,1:6));

y = -pinvJb*Jc(:,7:end)*qD;

== matlab function DesValues/State Machine/w_H_root_link4/fromImuToHomogeousTransformFCN ==
  data: imu_H_link input double; imu_H_link_0 input double; link_H_root input double; inertial_0 input double; inertial input double; neck input double; w_H_root output double; CONFIG parameter double
function w_H_root = fromBaseToWorldWithImuFCN(imu_H_link,imu_H_link_0,link_H_root,inertial_0,inertial,neck,CONFIG)
%#codegen
w_H_root = fromBaseToWorldWithImu(imu_H_link,imu_H_link_0,link_H_root,inertial_0,inertial,neck,CONFIG);

== matlab function DesValues/State Machine/w_H_root_link1/fromImuToHomogeousTransformFCN ==
  data: imu_H_link input double; imu_H_link_0 input double; link_H_root input double; inertial_0 input double; inertial input double; neck input double; w_H_root output double; CONFIG parameter double
function w_H_root = fromBaseToWorldWithImuFCN(imu_H_link,imu_H_link_0,link_H_root,inertial_0,inertial,neck,CONFIG)
%#codegen
w_H_root = fromBaseToWorldWithImu(imu_H_link,imu_H_link_0,link_H_root,inertial_0,inertial,neck,CONFIG);

== matlab function DesValues/Internal coordinator/refGen/refGenFCN ==
  data: xCom0 input double; qDes output double; q0 input double; t input double; references parameter double; desired_x_dx_ddx_CoM output double
function [qDes,desired_x_dx_ddx_CoM] = refGenFCN(xCom0,q0,t,references)
%#codegen

[qDes,desired_x_dx_ddx_CoM] = refGen(xCom0,q0,t,references);

== matlab function DesValues/State Machine Walking/w_H_root_link4/fromImuToHomogeousTransformFCN ==
  data: imu_H_link input double; imu_H_link_0 input double; link_H_root input double; inertial_0 input double; inertial input double; neck input double; w_H_root output double; CONFIG parameter double
function w_H_root = fromBaseToWorldWithImuFCN(imu_H_link,imu_H_link_0,link_H_root,inertial_0,inertial,neck,CONFIG)
%#codegen
w_H_root = fromBaseToWorldWithImu(imu_H_link,imu_H_link_0,link_H_root,inertial_0,inertial,neck,CONFIG);

== matlab function DesValues/State Machine/nu/MATLAB Function ==
  data: JcLeftFoot input double; JcRightFoot input double; activeFeetConstraints input double; y output double; qD input double; reg parameter double
function y = fcn(JcLeftFoot,JcRightFoot,activeFeetConstraints,qD,reg)
%#codegen

Jc = [activeFeetConstraints(1)*JcLeftFoot;
      activeFeetConstraints(2)*JcRightFoot];

pinvJb = pinvDamped(Jc(:,1:6),reg.pinvDampVb);  
  
% pinvJb = pinv(Jc(:,1:6));

y = -pinvJb*Jc(:,7:end)*qD;

== matlab function DesValues/State Machine/stateMachineFCN ==
  data: wrench_rightFoot input double; wrench_leftFoot input double; w_H_b output double; CoMDes output double; qDes output double; constraints output double; CoM_0 input double; q0 input double; l_sole_CoM input double; r_sole_CoM input double; qj input double; t input double; l_sole_H_b input double; r_sole_H_b input double; sm parameter double; impedances output double; kpCom output double; kdCom output double; gain parameter double; currentState output double; jointsSmoothingTime output double
function [w_H_b, CoMDes,qDes,constraints,impedances,kpCom,kdCom,currentState,jointsSmoothingTime] = ...
    stateMachineFCN(wrench_rightFoot,wrench_leftFoot,CoM_0, q0, l_sole_CoM,r_sole_CoM,qj, t, l_sole_H_b, r_sole_H_b, sm,gain)
%#codegen
 
[w_H_b, CoMDes,qDes,constraints,impedances,kpCom,kdCom,currentState,jointsSmoothingTime] = ...
    stateMachine(CoM_0, q0, l_sole_CoM,r_sole_CoM,qj, t, wrench_rightFoot,wrench_leftFoot,l_sole_H_b, r_sole_H_b, sm,gain);

== matlab function DesValues/State Machine Walking/w_H_root_link1/fromImuToHomogeousTransformFCN ==
  data: imu_H_link input double; imu_H_link_0 input double; link_H_root input double; inertial_0 input double; inertial input double; neck input double; w_H_root output double; CONFIG parameter double
function w_H_root = fromBaseToWorldWithImuFCN(imu_H_link,imu_H_link_0,link_H_root,inertial_0,inertial,neck,CONFIG)
%#codegen
w_H_root = fromBaseToWorldWithImu(imu_H_link,imu_H_link_0,link_H_root,inertial_0,inertial,neck,CONFIG);

== matlab function Dump and visualize/plotNorms/norm ==
  data: u input double; normU output double
function normU = fcn(u)
%#codegen

normU = norm(u);

== matlab function Dump and visualize/plotNorms/norm1 ==
  data: u input double; normU output double
function normU = fcn(u)
%#codegen

normU = norm(u);

== matlab function controller_QP/tau(f)  ==
  data: tauModel output double; Sigma output double; NA output double; fHdotDesC1C2 output double; HessianMatrixQP1Foot output double; gradientQP1Foot output double; ConstraintsMatrixQP1Foot output double; bVectorConstraintsQp1Foot output double; HessianMatrixQP2Feet output double; gradientQP2Feet output double; ConstraintsMatrixQP2Feet output double; bVectorConstraintsQp2Feet output double; constraints input double; ROBOT_DOF_FOR_SIMULINK input double; ConstraintsMatrix input double; bVectorConstraints input double; q input double; qDes input double; v input double; M input double; h input double; H input double; intHw input double; w_H_l_sole input double; w_H_r_sole input double; JL input double; JR input double; dJLv input double; dJRv input double; xcom input double; J_CoM input double; desired_x_dx_ddx_CoM input double; gainsPCOM input double; gainsDCOM input double; impedances input double; intErrorCoM input double; ki_int_qtilde input double; reg parameter double; gain parameter double; errorCoM output double; qTilde output double; f output double
function [tauModel,Sigma,NA,fHdotDesC1C2, ...
          HessianMatrixQP1Foot,gradientQP1Foot,ConstraintsMatrixQP1Foot,bVectorConstraintsQp1Foot,...
          HessianMatrixQP2Feet,gradientQP2Feet,ConstraintsMatrixQP2Feet,bVectorConstraintsQp2Feet,...
          errorCoM,qTilde,f]    =  ...
          balancingControllerFCN(constraints,ROBOT_DOF_FOR_SIMULINK,ConstraintsMatrix,bVectorConstraints,...
          q,qDes,v, M, h , H,intHw,w_H_l_sole, w_H_r_sole, JL,JR, dJLv,dJRv, xcom,J_CoM, desired_x_dx_ddx_CoM,...
          gainsPCOM,gainsDCOM,impedances, intErrorCoM,ki_int_qtilde,reg,gain)
%#codegen
    [tauModel,Sigma,NA,fHdotDesC1C2, ...
                  HessianMatrixQP1Foot,gradientQP1Foot,ConstraintsMatrixQP1Foot,bVectorConstraintsQp1Foot,...
                  HessianMatrixQP2Feet,gradientQP2Feet,ConstraintsMatrixQP2Feet,bVectorConstraintsQp2Feet,...
                  errorCoM,qTilde,f]    =  ...
                  balancingController(constraints,ROBOT_DOF_FOR_SIMULINK,ConstraintsMatrix,bVectorConstraints,...
                  q,qDes,v, M, h , H,intHw,w_H_l_sole, w_H_r_sole, JL,JR, dJLv,dJRv, xcom,J_CoM, desired_x_dx_ddx_CoM,...
                  gainsPCOM,gainsDCOM,impedances,intErrorCoM,ki_int_qtilde,reg,gain);
end

== matlab function emergency stop: joint limits/MATLAB Function ==
  data: umin input double; umax input double; u input double; inRange output double; tol input double
function inRange = checkRange(umin, umax, u, tol)
%#codegen

res = u < umin + tol | u > umax - tol;
res = sum(res);
if res==0
    inRange = 1;
else
    inRange = 0;
    u < umin + tol | u > umax - tol
end

== matlab function DesValues/State Machine Step Recovery/nu/MATLAB Function ==
  data: JcLeftFoot input double; JcRightFoot input double; activeFeetConstraints input double; y output double; qD input double; reg parameter double
function y = fcn(JcLeftFoot,JcRightFoot,activeFeetConstraints,qD,reg)
%#codegen

Jc = [activeFeetConstraints(1)*JcLeftFoot;
      activeFeetConstraints(2)*JcRightFoot];

pinvJb = pinvDamped(Jc(:,1:6),reg.pinvDampVb);  
  
% pinvJb = pinv(Jc(:,1:6));

y = -pinvJb*Jc(:,7:end)*qD;

== matlab function controller_QP/integralOf Hw/MATLAB Function1 ==
  data: H input double; deltaPhi output double
function deltaPhi = generateCentroidalOrient(H)
%#codegen

deltaPhi = H(4:end);

end

== matlab function DesValues/State Machine/visualise inertial/Visualize hom transf1/MATLAB Function ==
  data: R input double; rollPitchYaw output double
function rollPitchYaw = buildHomogenousTranformation(R)
%#codegen

rollPitchYaw = rollPitchYawFromRotation(R);

rollPitchYaw = rollPitchYaw*180/pi;

== matlab function DesValues/State Machine/visualise inertial/Visualize hom transf2/MATLAB Function ==
  data: R input double; rollPitchYaw output double
function rollPitchYaw = buildHomogenousTranformation(R)
%#codegen

rollPitchYaw = rollPitchYawFromRotation(R);

rollPitchYaw = rollPitchYaw*180/pi;

== matlab function DesValues/State Machine/visualise inertial/Visualize hom transf4/MATLAB Function ==
  data: R input double; rollPitchYaw output double
function rollPitchYaw = buildHomogenousTranformation(R)
%#codegen

rollPitchYaw = rollPitchYawFromRotation(R);

rollPitchYaw = rollPitchYaw*180/pi;

== matlab function DesValues/State Machine/visualise inertial/Visualize hom transf5/MATLAB Function ==
  data: R input double; rollPitchYaw output double
function rollPitchYaw = buildHomogenousTranformation(R)
%#codegen

rollPitchYaw = rollPitchYawFromRotation(R);

rollPitchYaw = rollPitchYaw*180/pi;

== matlab function DesValues/State Machine/visualise inertial/Visualize hom transf6/MATLAB Function ==
  data: R input double; rollPitchYaw output double
function rollPitchYaw = buildHomogenousTranformation(R)
%#codegen

rollPitchYaw = rollPitchYawFromRotation(R);

rollPitchYaw = rollPitchYaw*180/pi;

== matlab function DesValues/State Machine/visualise inertial/Visualize hom transf3/MATLAB Function ==
  data: R input double; rollPitchYaw output double
function rollPitchYaw = buildHomogenousTranformation(R)
%#codegen

rollPitchYaw = rollPitchYawFromRotation(R);

rollPitchYaw = rollPitchYaw*180/pi;

== matlab function DesValues/State Machine/visualise inertial/w_H_root_link4/fromImuToHomogeousTransformFCN ==
  data: imu_H_link input double; imu_H_link_0 input double; link_H_root input double; inertial_0 input double; inertial input double; neck input double; w_H_root output double; CONFIG parameter double
function w_H_root = fromBaseToWorldWithImuFCN(imu_H_link,imu_H_link_0,link_H_root,inertial_0,inertial,neck,CONFIG)
%#codegen
w_H_root = fromBaseToWorldWithImu(imu_H_link,imu_H_link_0,link_H_root,inertial_0,inertial,neck,CONFIG);

== matlab function DesValues/State Machine Step Recovery/stateMachineFCN ==
  data: wrench_rightFoot input double; wrench_leftFoot input double; w_H_b output double; CoMDes output double; qDes output double; constraints output double; CoM_0 input double; q0 input double; l_sole_CoM input double; r_sole_CoM input double; qj input double; t input double; l_sole_H_b input double; r_sole_H_b input double; sm parameter double; impedances output double; kpCom output double; kdCom output double; gain parameter double; currentState output double; jointsSmoothingTime output double; STEP_DOWN input double; COM_l_v input double; r_CxP input double; MAKE_A_STEP input double; QP_OFF output double; SMOOTH output double; SMOOTH_com output double; q_step_legs input double; COM_ref input double; l_solex input double; r_solex input double
function [w_H_b, CoMDes,qDes,constraints,impedances,kpCom,kdCom,currentState,jointsSmoothingTime, QP_OFF, SMOOTH, SMOOTH_com] = ...
    stateMachineFCN(wrench_rightFoot,wrench_leftFoot,CoM_0, q0, l_sole_CoM,r_sole_CoM,qj, t, l_sole_H_b, r_sole_H_b, sm,gain, STEP_DOWN, COM_l_v, r_CxP, MAKE_A_STEP, q_step_legs, COM_ref, l_solex, r_solex)
%#codegen
 
[w_H_b, CoMDes,qDes,constraints,impedances,kpCom,kdCom,currentState,jointsSmoothingTime, QP_OFF, SMOOTH, SMOOTH_com] = ...
    stateMachineStep(CoM_0, q0, l_sole_CoM,r_sole_CoM,qj, t, wrench_rightFoot,wrench_leftFoot,l_sole_H_b, r_sole_H_b, sm,gain, STEP_DOWN, r_CxP, COM_l_v, MAKE_A_STEP, q_step_legs, COM_ref, l_solex, r_solex);

== matlab function DesValues/State Machine Step Recovery/visualise inertial/Visualize hom transf1/MATLAB Function ==
  data: R input double; rollPitchYaw output double
function rollPitchYaw = buildHomogenousTranformation(R)
%#codegen

rollPitchYaw = rollPitchYawFromRotation(R);

rollPitchYaw = rollPitchYaw*180/pi;

== matlab function DesValues/State Machine Step Recovery/visualise inertial/Visualize hom transf2/MATLAB Function ==
  data: R input double; rollPitchYaw output double
function rollPitchYaw = buildHomogenousTranformation(R)
%#codegen

rollPitchYaw = rollPitchYawFromRotation(R);

rollPitchYaw = rollPitchYaw*180/pi;

== matlab function DesValues/State Machine Step Recovery/visualise inertial/Visualize hom transf3/MATLAB Function ==
  data: R input double; rollPitchYaw output double
function rollPitchYaw = buildHomogenousTranformation(R)
%#codegen

rollPitchYaw = rollPitchYawFromRotation(R);

rollPitchYaw = rollPitchYaw*180/pi;

== matlab function DesValues/State Machine Step Recovery/visualise inertial/Visualize hom transf4/MATLAB Function ==
  data: R input double; rollPitchYaw output double
function rollPitchYaw = buildHomogenousTranformation(R)
%#codegen

rollPitchYaw = rollPitchYawFromRotation(R);

rollPitchYaw = rollPitchYaw*180/pi;

== matlab function DesValues/State Machine Step Recovery/visualise inertial/Visualize hom transf5/MATLAB Function ==
  data: R input double; rollPitchYaw output double
function rollPitchYaw = buildHomogenousTranformation(R)
%#codegen

rollPitchYaw = rollPitchYawFromRotation(R);

rollPitchYaw = rollPitchYaw*180/pi;
